simulink library "inp"  (R2021b)
settings: Solver=VariableStepAuto  StartTime=0.0  StopTime=10.0  RelTol=1e-3
undefined symbols (not defined in the file): C_TASK_5MS_S, FALSE, KINP_AcoreReadyToSlp_flg_ovrdflg, KINP_AcoreReadyToSlp_flg_ovrdval, KINP_AllowMovThd_OTA_enum_ovrdflg, KINP_AllowMovThd_OTA_enum_ovrdval, KINP_APSAngleTarget_Deg_ovrdflg, KINP_APSAngleTarget_Deg_ovrdval, KINP_APSDecReq_mps2_ovrdflg, KINP_APSDecReq_mps2_ovrdval, KINP_APSDecReqA_flg_ovrdflg, KINP_APSDecReqA_flg_ovrdval, KINP_APSDFLL_cm_ovrdflg, KINP_APSDFLL_cm_ovrdval, KINP_APSDFLR_cm_ovrdflg, KINP_APSDFLR_cm_ovrdval, KINP_APSDRLL_cm_ovrdflg, KINP_APSDRLL_cm_ovrdval, KINP_APSDRLR_cm_ovrdflg, KINP_APSDRLR_cm_ovrdval, KINP_APSExitCondition_enum_ovrdflg, KINP_APSExitCondition_enum_ovrdval, KINP_APSHWVer_enum_ovrdflg, KINP_APSHWVer_enum_ovrdval, KINP_APSProgressPCT_pct_ovrdflg, KINP_APSProgressPCT_pct_ovrdval, KINP_APSPwrReq_enum_ovrdflg, KINP_APSPwrReq_enum_ovrdval, KINP_APSReq_enum_ovrdflg, KINP_APSReq_enum_ovrdval, KINP_APSRQDisplay_enum_ovrdflg, KINP_APSRQDisplay_enum_ovrdval, KINP_APSRqEPASCtrl_flg_ovrdflg, KINP_APSRqEPASCtrl_flg_ovrdval, KINP_APSShiftPosnReq_enum_ovrdval, KINP_APSShiftPosnReq_enum_ovrflg, KINP_APSSpeedCMD_kph_ovrdval, KINP_APSSpeedCMD_kph_ovrflg, KINP_APSStaSystem_enum_ovrdflg, KINP_APSStaSystem_enum_ovrdval, KINP_APSSWVer_enum_ovrdflg, KINP_APSSWVer_enum_ovrdval, KINP_APSVMCReqA_flg_ovrdval, KINP_APSVMCReqA_flg_ovrflg, KINP_APSVRqEPASCtrl_flg_ovrdflg, KINP_APSVRqEPASCtrl_flg_ovrdval, KINP_AuxBattVolmV_mV_ovrdflg, KINP_AuxBattVolmV_mV_ovrdval, KINP_CAASSta_enum_ovrdflg, KINP_CAASSta_enum_ovrdval, KINP_CAASVMCReqA_flg_ovrdval, KINP_CAASVMCReqA_flg_ovrflg, KINP_CAN1BusOff_flg_ovrdflg, KINP_CAN1BusOff_flg_ovrdval, KINP_CAN2BusOff_flg_ovrdflg, KINP_CAN2BusOff_flg_ovrdval, KINP_CAN3BusOff_flg_ovrdflg, KINP_CAN3BusOff_flg_ovrdval, KINP_CAN4BusOff_flg_ovrdflg, KINP_CAN4BusOff_flg_ovrdval ... (+152)
libraries: FVT_lib x1035, hcu_lib x1
(part 11 of 33)

== system inp/INP/CAN6/CreateBus ==
  inp_CanValid_bus : Inport
  inp_Hal_bus : Inport  Port=2
  UnitConverter_{1..5,14..15,21,23..25,27,42,45..46,52,54,56..60,62..64,67..68,86..87,90,93,96..97} (33 alike) : DataTypeConversion  OutDataTypeStr=boolean
  UnitConverter_{6..10,12..13,35..36,50,70..85,88..89,91..92} (30 alike) : DataTypeConversion  OutDataTypeStr=single
  UnitConverter_{11,16..20,22,26,28..34,37..41,43..44,47..49,51,53,55,61,65..66,69,94..95,98..99} (36 alike) : DataTypeConversion  OutDataTypeStr=uint8
  bus_creator : BusCreator  Inputs=99
  bus_selector : BusSelector  OutputSignals=VINP_CANMsgValidFCM1_flg,VINP_CANMsgValidFCM2_flg,VINP_CANMsgValidFCM3_flg,VINP_CANMsgValidFCM4_flg,VINP_CANMsgValidSRR1_flg
  bus_selector_1 : BusSelector  OutputSignals=VINP_ACCComfortBandLower_mps2,VINP_ACCComfortBandUpper_mps2,VINP_ACCJerkLowerLimit_mps3,VINP_ACCJerkUpperLimit_mps3,VINP_ACCObjDist_m,VINP_ACCObjDstLvl_enum,VINP_ACCObjRelSpd_mps,VINP_ACCRequiredAccel_mps2,VINP_ACCTakeoverReq_flg,VINP_ACCVehHoldReq_flg,VINP_ADASACCSta_enum,VINP_ADASAEBReq_enum,VINP_ADASAEBSta_enum,VINP_ADASCAMSpdLim_enum,VINP_ADASDBSReq_enum,VINP_ADASFCWMute_flg,VINP_ADASFCWSta_enum,VINP_ADASFaultSta_flg,VINP_ADASFltWrnReq_flg,VINP_ADASForceIdle_flg,VINP_ADASISASta_enum,VINP_ADASLDWMute_flg,VINP_ADASLDWSta_enum,VINP_ADASLFCHandsOffWarning_enum,VINP_ADASLFCSta_enum,VINP_ADASLFCWarnSound_enum,VINP_ADASLKASta_enum,VINP_ADASLaneModeL_enum,VINP_ADASLaneModeR_enum,VINP_ADASLanecurveL_raw32,VINP_ADASLanecurveR_raw32,VINP_ADASLanetypeL_enum,VINP_ADASLanetypeR_enum,VINP_ADASSLIFSpdLim_enum,VINP_ADASSLIFSta_enum,VINP_ADASShftPosnReq_enum,VINP_ADASShftPosnReqA_flg,VINP_ADASVehSpdLim_enum,VINP_ADASWarningMsg_enum,VINP_AEBVehHoldReq_flg,VINP_CameraBlockage_flg,VINP_FCM1Checksum_enum,VINP_FCM1LifeCount_enum,VINP_FCMACCmode_enum,VINP_FCMLKAStrToqReq_Nm,VINP_FCMLKATOIAct_enum,VINP_FCMLKATOIFault_flg,VINP_ForceLowBeam_enum,VINP_HazardWarningReq_flg,VINP_ISAWarningMsg_enum,VINP_LKAHODDisplayWarning_flg,VINP_LKAHODSoundWarning_flg,VINP_LVDAACCStatusInformation_flg,VINP_LVDADisabled_flg,VINP_LVDAFailinfo_flg,VINP_LVDAMuteSta_enum,VINP_LVDAWarning_flg,VINP_LeftTurnLightReq_flg,VINP_RightTurnLightReq_flg,VINP_TargetType_enum,VINP_TimeGapLevel_enum,VINP_FCM2CSErr_flg,VINP_FCM2RCErr_flg,VINP_ADBVehDst1Val_enum,VINP_MELaneCurvDervLt_raw32,VINP_MELaneCurvDervLt2_raw32,VINP_MELaneCurvDervRt_raw32,VINP_MELaneCurvDervRt2_raw32,VINP_MELaneCurvLt_raw32,VINP_MELaneCurvLt2_raw32,VINP_MELaneCurvRt_raw32,VINP_MELaneCurvRt2_raw32,VINP_MELaneHeadAngLt_radians,VINP_MELaneHeadAngLt2_radians,VINP_MELaneHeadAngRt_radians,VINP_MELaneHeadAngRt2_radians,VINP_MELanePosLt_m,VINP_MELanePosLt2_m,VINP_MELanePosRt_m,VINP_MELanePosRt2_m,VINP_FCM4CSErr_flg,VINP_FCM4RCErr_flg,VINP_ADASAngCtrlTqWeightGain_pct,VINP_ADASDesStrWhlAngCtrlCmd_Deg,VINP_ADASDrvInputTqBoostAct_flg,VINP_ADASDrvInputTqBoostGain_pct,VINP_ADASMaxAngCtrlOutTqLimit_Nm,VINP_ADASStrWhlAngCtrlStatus_flg,VINP_SRRBSDWarnL_enum,VINP_SRRBSDWarnR_enum,VINP_SRRODASoundL_flg,VINP_SRRODASoundR_flg,VINP_SRRODAWarnL_enum,VINP_SRRODAWarnR_enum
  BINP_outputs : Outport
  wires:
  inp_CanValid_bus/1 -> [inp_CanValid_bus]
  inp_Hal_bus/1 -> [inp_Hal_bus]
  bus_selector/1 -> UnitConverter_1/1  "<VINP_CANMsgValidFCM1_flg>"
  UnitConverter_1/1 -> bus_creator/1  "VINP_CANMsgValidFCM1_flg"
  bus_selector/2 -> UnitConverter_2/1  "<VINP_CANMsgValidFCM2_flg>"
  UnitConverter_2/1 -> bus_creator/2  "VINP_CANMsgValidFCM2_flg"
  bus_selector/3 -> UnitConverter_3/1  "<VINP_CANMsgValidFCM3_flg>"
  UnitConverter_3/1 -> bus_creator/3  "VINP_CANMsgValidFCM3_flg"
  bus_selector/4 -> UnitConverter_4/1  "<VINP_CANMsgValidFCM4_flg>"
  UnitConverter_4/1 -> bus_creator/4  "VINP_CANMsgValidFCM4_flg"
  bus_selector/5 -> UnitConverter_5/1  "<VINP_CANMsgValidSRR1_flg>"
  UnitConverter_5/1 -> bus_creator/5  "VINP_CANMsgValidSRR1_flg"
  bus_selector_1/1 -> UnitConverter_6/1  "<VINP_ACCComfortBandLower_mps2>"
  UnitConverter_6/1 -> bus_creator/6  "VINP_ACCComfortBandLower_mps2"
  bus_selector_1/2 -> UnitConverter_7/1  "<VINP_ACCComfortBandUpper_mps2>"
  UnitConverter_7/1 -> bus_creator/7  "VINP_ACCComfortBandUpper_mps2"
  bus_selector_1/3 -> UnitConverter_8/1  "<VINP_ACCJerkLowerLimit_mps3>"
  UnitConverter_8/1 -> bus_creator/8  "VINP_ACCJerkLowerLimit_mps3"
  bus_selector_1/4 -> UnitConverter_9/1  "<VINP_ACCJerkUpperLimit_mps3>"
  UnitConverter_9/1 -> bus_creator/9  "VINP_ACCJerkUpperLimit_mps3"
  bus_selector_1/5 -> UnitConverter_10/1  "<VINP_ACCObjDist_m>"
  UnitConverter_10/1 -> bus_creator/10  "VINP_ACCObjDist_m"
  bus_selector_1/6 -> UnitConverter_11/1  "<VINP_ACCObjDstLvl_enum>"
  UnitConverter_11/1 -> bus_creator/11  "VINP_ACCObjDstLvl_enum"
  bus_selector_1/7 -> UnitConverter_12/1  "<VINP_ACCObjRelSpd_mps>"
  UnitConverter_12/1 -> bus_creator/12  "VINP_ACCObjRelSpd_mps"
  bus_selector_1/8 -> UnitConverter_13/1  "<VINP_ACCRequiredAccel_mps2>"
  UnitConverter_13/1 -> bus_creator/13  "VINP_ACCRequiredAccel_mps2"
  bus_selector_1/9 -> UnitConverter_14/1  "<VINP_ACCTakeoverReq_flg>"
  UnitConverter_14/1 -> bus_creator/14  "VINP_ACCTakeoverReq_flg"
  bus_selector_1/10 -> UnitConverter_15/1  "<VINP_ACCVehHoldReq_flg>"
  UnitConverter_15/1 -> bus_creator/15  "VINP_ACCVehHoldReq_flg"
  bus_selector_1/11 -> UnitConverter_16/1  "<VINP_ADASACCSta_enum>"
  UnitConverter_16/1 -> bus_creator/16  "VINP_ADASACCSta_enum"
  bus_selector_1/12 -> UnitConverter_17/1  "<VINP_ADASAEBReq_enum>"
  UnitConverter_17/1 -> bus_creator/17  "VINP_ADASAEBReq_enum"
  bus_selector_1/13 -> UnitConverter_18/1  "<VINP_ADASAEBSta_enum>"
  UnitConverter_18/1 -> bus_creator/18  "VINP_ADASAEBSta_enum"
  bus_selector_1/14 -> UnitConverter_19/1  "<VINP_ADASCAMSpdLim_enum>"
  UnitConverter_19/1 -> bus_creator/19  "VINP_ADASCAMSpdLim_enum"
  bus_selector_1/15 -> UnitConverter_20/1  "<VINP_ADASDBSReq_enum>"
  UnitConverter_20/1 -> bus_creator/20  "VINP_ADASDBSReq_enum"
  bus_selector_1/16 -> UnitConverter_21/1  "<VINP_ADASFCWMute_flg>"
  UnitConverter_21/1 -> bus_creator/21  "VINP_ADASFCWMute_flg"
  bus_selector_1/17 -> UnitConverter_22/1  "<VINP_ADASFCWSta_enum>"
  UnitConverter_22/1 -> bus_creator/22  "VINP_ADASFCWSta_enum"
  bus_selector_1/18 -> UnitConverter_23/1  "<VINP_ADASFaultSta_flg>"
  UnitConverter_23/1 -> bus_creator/23  "VINP_ADASFaultSta_flg"
  bus_selector_1/19 -> UnitConverter_24/1  "<VINP_ADASFltWrnReq_flg>"
  UnitConverter_24/1 -> bus_creator/24  "VINP_ADASFltWrnReq_flg"
  bus_selector_1/20 -> UnitConverter_25/1  "<VINP_ADASForceIdle_flg>"
  UnitConverter_25/1 -> bus_creator/25  "VINP_ADASForceIdle_flg"
  bus_selector_1/21 -> UnitConverter_26/1  "<VINP_ADASISASta_enum>"
  UnitConverter_26/1 -> bus_creator/26  "VINP_ADASISASta_enum"
  bus_selector_1/22 -> UnitConverter_27/1  "<VINP_ADASLDWMute_flg>"
  UnitConverter_27/1 -> bus_creator/27  "VINP_ADASLDWMute_flg"
  bus_selector_1/23 -> UnitConverter_28/1  "<VINP_ADASLDWSta_enum>"
  UnitConverter_28/1 -> bus_creator/28  "VINP_ADASLDWSta_enum"
  bus_selector_1/24 -> UnitConverter_29/1  "<VINP_ADASLFCHandsOffWarning_enum>"
  UnitConverter_29/1 -> bus_creator/29  "VINP_ADASLFCHandsOffWarning_enum"
  bus_selector_1/25 -> UnitConverter_30/1  "<VINP_ADASLFCSta_enum>"
  UnitConverter_30/1 -> bus_creator/30  "VINP_ADASLFCSta_enum"
  bus_selector_1/26 -> UnitConverter_31/1  "<VINP_ADASLFCWarnSound_enum>"
  UnitConverter_31/1 -> bus_creator/31  "VINP_ADASLFCWarnSound_enum"
  bus_selector_1/27 -> UnitConverter_32/1  "<VINP_ADASLKASta_enum>"
  UnitConverter_32/1 -> bus_creator/32  "VINP_ADASLKASta_enum"
  bus_selector_1/28 -> UnitConverter_33/1  "<VINP_ADASLaneModeL_enum>"
  UnitConverter_33/1 -> bus_creator/33  "VINP_ADASLaneModeL_enum"
  bus_selector_1/29 -> UnitConverter_34/1  "<VINP_ADASLaneModeR_enum>"
  UnitConverter_34/1 -> bus_creator/34  "VINP_ADASLaneModeR_enum"
  bus_selector_1/30 -> UnitConverter_35/1  "<VINP_ADASLanecurveL_raw32>"
  UnitConverter_35/1 -> bus_creator/35  "VINP_ADASLanecurveL_raw32"
  bus_selector_1/31 -> UnitConverter_36/1  "<VINP_ADASLanecurveR_raw32>"
  UnitConverter_36/1 -> bus_creator/36  "VINP_ADASLanecurveR_raw32"
  bus_selector_1/32 -> UnitConverter_37/1  "<VINP_ADASLanetypeL_enum>"
  UnitConverter_37/1 -> bus_creator/37  "VINP_ADASLanetypeL_enum"
  bus_selector_1/33 -> UnitConverter_38/1  "<VINP_ADASLanetypeR_enum>"
  UnitConverter_38/1 -> bus_creator/38  "VINP_ADASLanetypeR_enum"
  bus_selector_1/34 -> UnitConverter_39/1  "<VINP_ADASSLIFSpdLim_enum>"
  UnitConverter_39/1 -> bus_creator/39  "VINP_ADASSLIFSpdLim_enum"
  bus_selector_1/35 -> UnitConverter_40/1  "<VINP_ADASSLIFSta_enum>"
  UnitConverter_40/1 -> bus_creator/40  "VINP_ADASSLIFSta_enum"
  bus_selector_1/36 -> UnitConverter_41/1  "<VINP_ADASShftPosnReq_enum>"
  UnitConverter_41/1 -> bus_creator/41  "VINP_ADASShftPosnReq_enum"
  bus_selector_1/37 -> UnitConverter_42/1  "<VINP_ADASShftPosnReqA_flg>"
  UnitConverter_42/1 -> bus_creator/42  "VINP_ADASShftPosnReqA_flg"
  bus_selector_1/38 -> UnitConverter_43/1  "<VINP_ADASVehSpdLim_enum>"
  UnitConverter_43/1 -> bus_creator/43  "VINP_ADASVehSpdLim_enum"
  bus_selector_1/39 -> UnitConverter_44/1  "<VINP_ADASWarningMsg_enum>"
  UnitConverter_44/1 -> bus_creator/44  "VINP_ADASWarningMsg_enum"
  bus_selector_1/40 -> UnitConverter_45/1  "<VINP_AEBVehHoldReq_flg>"
  UnitConverter_45/1 -> bus_creator/45  "VINP_AEBVehHoldReq_flg"
  bus_selector_1/41 -> UnitConverter_46/1  "<VINP_CameraBlockage_flg>"
  UnitConverter_46/1 -> bus_creator/46  "VINP_CameraBlockage_flg"
  bus_selector_1/42 -> UnitConverter_47/1  "<VINP_FCM1Checksum_enum>"
  UnitConverter_47/1 -> bus_creator/47  "VINP_FCM1Checksum_enum"
  bus_selector_1/43 -> UnitConverter_48/1  "<VINP_FCM1LifeCount_enum>"
  UnitConverter_48/1 -> bus_creator/48  "VINP_FCM1LifeCount_enum"
  bus_selector_1/44 -> UnitConverter_49/1  "<VINP_FCMACCmode_enum>"
  UnitConverter_49/1 -> bus_creator/49  "VINP_FCMACCmode_enum"
  bus_selector_1/45 -> UnitConverter_50/1  "<VINP_FCMLKAStrToqReq_Nm>"
  UnitConverter_50/1 -> bus_creator/50  "VINP_FCMLKAStrToqReq_Nm"
  bus_selector_1/46 -> UnitConverter_51/1  "<VINP_FCMLKATOIAct_enum>"
  UnitConverter_51/1 -> bus_creator/51  "VINP_FCMLKATOIAct_enum"
  bus_selector_1/47 -> UnitConverter_52/1  "<VINP_FCMLKATOIFault_flg>"
  UnitConverter_52/1 -> bus_creator/52  "VINP_FCMLKATOIFault_flg"
  bus_selector_1/48 -> UnitConverter_53/1  "<VINP_ForceLowBeam_enum>"
  UnitConverter_53/1 -> bus_creator/53  "VINP_ForceLowBeam_enum"
  bus_selector_1/49 -> UnitConverter_54/1  "<VINP_HazardWarningReq_flg>"
  UnitConverter_54/1 -> bus_creator/54  "VINP_HazardWarningReq_flg"
  bus_selector_1/50 -> UnitConverter_55/1  "<VINP_ISAWarningMsg_enum>"
  UnitConverter_55/1 -> bus_creator/55  "VINP_ISAWarningMsg_enum"
  bus_selector_1/51 -> UnitConverter_56/1  "<VINP_LKAHODDisplayWarning_flg>"
  UnitConverter_56/1 -> bus_creator/56  "VINP_LKAHODDisplayWarning_flg"
  bus_selector_1/52 -> UnitConverter_57/1  "<VINP_LKAHODSoundWarning_flg>"
  UnitConverter_57/1 -> bus_creator/57  "VINP_LKAHODSoundWarning_flg"
  bus_selector_1/53 -> UnitConverter_58/1  "<VINP_LVDAACCStatusInformation_flg>"
  UnitConverter_58/1 -> bus_creator/58  "VINP_LVDAACCStatusInformation_flg"
  bus_selector_1/54 -> UnitConverter_59/1  "<VINP_LVDADisabled_flg>"
  UnitConverter_59/1 -> bus_creator/59  "VINP_LVDADisabled_flg"
  bus_selector_1/55 -> UnitConverter_60/1  "<VINP_LVDAFailinfo_flg>"
  UnitConverter_60/1 -> bus_creator/60  "VINP_LVDAFailinfo_flg"
  bus_selector_1/56 -> UnitConverter_61/1  "<VINP_LVDAMuteSta_enum>"
  UnitConverter_61/1 -> bus_creator/61  "VINP_LVDAMuteSta_enum"
  bus_selector_1/57 -> UnitConverter_62/1  "<VINP_LVDAWarning_flg>"
  UnitConverter_62/1 -> bus_creator/62  "VINP_LVDAWarning_flg"
  bus_selector_1/58 -> UnitConverter_63/1  "<VINP_LeftTurnLightReq_flg>"
  UnitConverter_63/1 -> bus_creator/63  "VINP_LeftTurnLightReq_flg"
  bus_selector_1/59 -> UnitConverter_64/1  "<VINP_RightTurnLightReq_flg>"
  UnitConverter_64/1 -> bus_creator/64  "VINP_RightTurnLightReq_flg"
  bus_selector_1/60 -> UnitConverter_65/1  "<VINP_TargetType_enum>"
  UnitConverter_65/1 -> bus_creator/65  "VINP_TargetType_enum"
  bus_selector_1/61 -> UnitConverter_66/1  "<VINP_TimeGapLevel_enum>"
  UnitConverter_66/1 -> bus_creator/66  "VINP_TimeGapLevel_enum"
  bus_selector_1/62 -> UnitConverter_67/1  "<VINP_FCM2CSErr_flg>"
  UnitConverter_67/1 -> bus_creator/67  "VINP_FCM2CSErr_flg"
  bus_selector_1/63 -> UnitConverter_68/1  "<VINP_FCM2RCErr_flg>"
  UnitConverter_68/1 -> bus_creator/68  "VINP_FCM2RCErr_flg"
  bus_selector_1/64 -> UnitConverter_69/1  "<VINP_ADBVehDst1Val_enum>"
  UnitConverter_69/1 -> bus_creator/69  "VINP_ADBVehDst1Val_enum"
  bus_selector_1/65 -> UnitConverter_70/1  "<VINP_MELaneCurvDervLt_raw32>"
  UnitConverter_70/1 -> bus_creator/70  "VINP_MELaneCurvDervLt_raw32"
  bus_selector_1/66 -> UnitConverter_71/1  "<VINP_MELaneCurvDervLt2_raw32>"
  UnitConverter_71/1 -> bus_creator/71  "VINP_MELaneCurvDervLt2_raw32"
  bus_selector_1/67 -> UnitConverter_72/1  "<VINP_MELaneCurvDervRt_raw32>"
  UnitConverter_72/1 -> bus_creator/72  "VINP_MELaneCurvDervRt_raw32"
  bus_selector_1/68 -> UnitConverter_73/1  "<VINP_MELaneCurvDervRt2_raw32>"
  UnitConverter_73/1 -> bus_creator/73  "VINP_MELaneCurvDervRt2_raw32"
  bus_selector_1/69 -> UnitConverter_74/1  "<VINP_MELaneCurvLt_raw32>"
  UnitConverter_74/1 -> bus_creator/74  "VINP_MELaneCurvLt_raw32"
  bus_selector_1/70 -> UnitConverter_75/1  "<VINP_MELaneCurvLt2_raw32>"
  UnitConverter_75/1 -> bus_creator/75  "VINP_MELaneCurvLt2_raw32"
  bus_selector_1/71 -> UnitConverter_76/1  "<VINP_MELaneCurvRt_raw32>"
  UnitConverter_76/1 -> bus_creator/76  "VINP_MELaneCurvRt_raw32"
  bus_selector_1/72 -> UnitConverter_77/1  "<VINP_MELaneCurvRt2_raw32>"
  UnitConverter_77/1 -> bus_creator/77  "VINP_MELaneCurvRt2_raw32"
  bus_selector_1/73 -> UnitConverter_78/1  "<VINP_MELaneHeadAngLt_radians>"
  UnitConverter_78/1 -> bus_creator/78  "VINP_MELaneHeadAngLt_radians"
  bus_selector_1/74 -> UnitConverter_79/1  "<VINP_MELaneHeadAngLt2_radians>"
  UnitConverter_79/1 -> bus_creator/79  "VINP_MELaneHeadAngLt2_radians"
  bus_selector_1/75 -> UnitConverter_80/1  "<VINP_MELaneHeadAngRt_radians>"
  UnitConverter_80/1 -> bus_creator/80  "VINP_MELaneHeadAngRt_radians"
  bus_selector_1/76 -> UnitConverter_81/1  "<VINP_MELaneHeadAngRt2_radians>"
  UnitConverter_81/1 -> bus_creator/81  "VINP_MELaneHeadAngRt2_radians"
  bus_selector_1/77 -> UnitConverter_82/1  "<VINP_MELanePosLt_m>"
  UnitConverter_82/1 -> bus_creator/82  "VINP_MELanePosLt_m"
  bus_selector_1/78 -> UnitConverter_83/1  "<VINP_MELanePosLt2_m>"
  UnitConverter_83/1 -> bus_creator/83  "VINP_MELanePosLt2_m"
  bus_selector_1/79 -> UnitConverter_84/1  "<VINP_MELanePosRt_m>"
  UnitConverter_84/1 -> bus_creator/84  "VINP_MELanePosRt_m"
  bus_selector_1/80 -> UnitConverter_85/1  "<VINP_MELanePosRt2_m>"
  UnitConverter_85/1 -> bus_creator/85  "VINP_MELanePosRt2_m"
  bus_selector_1/81 -> UnitConverter_86/1  "<VINP_FCM4CSErr_flg>"
  UnitConverter_86/1 -> bus_creator/86  "VINP_FCM4CSErr_flg"
  bus_selector_1/82 -> UnitConverter_87/1  "<VINP_FCM4RCErr_flg>"
  UnitConverter_87/1 -> bus_creator/87  "VINP_FCM4RCErr_flg"
  bus_selector_1/83 -> UnitConverter_88/1  "<VINP_ADASAngCtrlTqWeightGain_pct>"
  UnitConverter_88/1 -> bus_creator/88  "VINP_ADASAngCtrlTqWeightGain_pct"
  bus_selector_1/84 -> UnitConverter_89/1  "<VINP_ADASDesStrWhlAngCtrlCmd_Deg>"
  UnitConverter_89/1 -> bus_creator/89  "VINP_ADASDesStrWhlAngCtrlCmd_Deg"
  bus_selector_1/85 -> UnitConverter_90/1  "<VINP_ADASDrvInputTqBoostAct_flg>"
  UnitConverter_90/1 -> bus_creator/90  "VINP_ADASDrvInputTqBoostAct_flg"
  bus_selector_1/86 -> UnitConverter_91/1  "<VINP_ADASDrvInputTqBoostGain_pct>"
  UnitConverter_91/1 -> bus_creator/91  "VINP_ADASDrvInputTqBoostGain_pct"
  bus_selector_1/87 -> UnitConverter_92/1  "<VINP_ADASMaxAngCtrlOutTqLimit_Nm>"
  UnitConverter_92/1 -> bus_creator/92  "VINP_ADASMaxAngCtrlOutTqLimit_Nm"
  bus_selector_1/88 -> UnitConverter_93/1  "<VINP_ADASStrWhlAngCtrlStatus_flg>"
  UnitConverter_93/1 -> bus_creator/93  "VINP_ADASStrWhlAngCtrlStatus_flg"
  bus_selector_1/89 -> UnitConverter_94/1  "<VINP_SRRBSDWarnL_enum>"
  UnitConverter_94/1 -> bus_creator/94  "VINP_SRRBSDWarnL_enum"
  bus_selector_1/90 -> UnitConverter_95/1  "<VINP_SRRBSDWarnR_enum>"
  UnitConverter_95/1 -> bus_creator/95  "VINP_SRRBSDWarnR_enum"
  bus_selector_1/91 -> UnitConverter_96/1  "<VINP_SRRODASoundL_flg>"
  UnitConverter_96/1 -> bus_creator/96  "VINP_SRRODASoundL_flg"
  bus_selector_1/92 -> UnitConverter_97/1  "<VINP_SRRODASoundR_flg>"
  UnitConverter_97/1 -> bus_creator/97  "VINP_SRRODASoundR_flg"
  bus_selector_1/93 -> UnitConverter_98/1  "<VINP_SRRODAWarnL_enum>"
  UnitConverter_98/1 -> bus_creator/98  "VINP_SRRODAWarnL_enum"
  bus_selector_1/94 -> UnitConverter_99/1  "<VINP_SRRODAWarnR_enum>"
  UnitConverter_99/1 -> bus_creator/99  "VINP_SRRODAWarnR_enum"
  [inp_CanValid_bus] -> bus_selector/1
  [inp_Hal_bus] -> bus_selector_1/1
  bus_creator/1 -> BINP_outputs/1

== system inp/INP/CAN6/SignalCheck ==
  inp_CanValid_bus : Inport
  TASK_TIME_S : Inport  Port=2
  BHAL_outputs : Inport  Port=3
  FCM1 : Subsystem
  FCM2 : Subsystem
  FCM3 : Subsystem
  FCM4 : Subsystem
  SRR1 : Subsystem
  bus_creator : BusCreator  Inputs=94
  inp_Hal_bus : Outport
  wires:
  inp_CanValid_bus/1 -> [inp_CanValid_bus]
  TASK_TIME_S/1 -> [TASK_TIME_S]
  BHAL_outputs/1 -> [BHAL_outputs]
  [BHAL_outputs] -> FCM1/1(BHAL_outputs)
  [inp_CanValid_bus] -> FCM1/2(inp_CanValid_bus)
  FCM1/1(VINP_ACCComfortBandLower_mps2) -> [VINP_ACCComfortBandLower_mps2]
  FCM1/2(VINP_ACCComfortBandUpper_mps2) -> [VINP_ACCComfortBandUpper_mps2]
  FCM1/3(VINP_ACCJerkLowerLimit_mps3) -> [VINP_ACCJerkLowerLimit_mps3]
  FCM1/4(VINP_ACCJerkUpperLimit_mps3) -> [VINP_ACCJerkUpperLimit_mps3]
  FCM1/5(VINP_ACCObjDist_m) -> [VINP_ACCObjDist_m]
  FCM1/6(VINP_ACCObjDstLvl_enum) -> [VINP_ACCObjDstLvl_enum]
  FCM1/7(VINP_ACCObjRelSpd_mps) -> [VINP_ACCObjRelSpd_mps]
  FCM1/8(VINP_ACCRequiredAccel_mps2) -> [VINP_ACCRequiredAccel_mps2]
  FCM1/9(VINP_ACCTakeoverReq_flg) -> [VINP_ACCTakeoverReq_flg]
  FCM1/10(VINP_ACCVehHoldReq_flg) -> [VINP_ACCVehHoldReq_flg]
  FCM1/11(VINP_ADASACCSta_enum) -> [VINP_ADASACCSta_enum]
  FCM1/12(VINP_ADASAEBReq_enum) -> [VINP_ADASAEBReq_enum]
  FCM1/13(VINP_ADASAEBSta_enum) -> [VINP_ADASAEBSta_enum]
  FCM1/14(VINP_ADASCAMSpdLim_enum) -> [VINP_ADASCAMSpdLim_enum]
  FCM1/15(VINP_ADASDBSReq_enum) -> [VINP_ADASDBSReq_enum]
  FCM1/16(VINP_ADASFCWMute_flg) -> [VINP_ADASFCWMute_flg]
  FCM1/17(VINP_ADASFCWSta_enum) -> [VINP_ADASFCWSta_enum]
  FCM1/18(VINP_ADASFaultSta_flg) -> [VINP_ADASFaultSta_flg]
  FCM1/19(VINP_ADASFltWrnReq_flg) -> [VINP_ADASFltWrnReq_flg]
  FCM1/20(VINP_ADASForceIdle_flg) -> [VINP_ADASForceIdle_flg]
  FCM1/21(VINP_ADASISASta_enum) -> [VINP_ADASISASta_enum]
  FCM1/22(VINP_ADASLDWMute_flg) -> [VINP_ADASLDWMute_flg]
  FCM1/23(VINP_ADASLDWSta_enum) -> [VINP_ADASLDWSta_enum]
  FCM1/24(VINP_ADASLFCHandsOffWarning_enum) -> [VINP_ADASLFCHandsOffWarning_enum]
  FCM1/25(VINP_ADASLFCSta_enum) -> [VINP_ADASLFCSta_enum]
  FCM1/26(VINP_ADASLFCWarnSound_enum) -> [VINP_ADASLFCWarnSound_enum]
  FCM1/27(VINP_ADASLKASta_enum) -> [VINP_ADASLKASta_enum]
  FCM1/28(VINP_ADASLaneModeL_enum) -> [VINP_ADASLaneModeL_enum]
  FCM1/29(VINP_ADASLaneModeR_enum) -> [VINP_ADASLaneModeR_enum]
  FCM1/30(VINP_ADASLanecurveL_raw32) -> [VINP_ADASLanecurveL_raw32]
  FCM1/31(VINP_ADASLanecurveR_raw32) -> [VINP_ADASLanecurveR_raw32]
  FCM1/32(VINP_ADASLanetypeL_enum) -> [VINP_ADASLanetypeL_enum]
  FCM1/33(VINP_ADASLanetypeR_enum) -> [VINP_ADASLanetypeR_enum]
  FCM1/34(VINP_ADASSLIFSpdLim_enum) -> [VINP_ADASSLIFSpdLim_enum]
  FCM1/35(VINP_ADASSLIFSta_enum) -> [VINP_ADASSLIFSta_enum]
  FCM1/36(VINP_ADASShftPosnReq_enum) -> [VINP_ADASShftPosnReq_enum]
  FCM1/37(VINP_ADASShftPosnReqA_flg) -> [VINP_ADASShftPosnReqA_flg]
  FCM1/38(VINP_ADASVehSpdLim_enum) -> [VINP_ADASVehSpdLim_enum]
  FCM1/39(VINP_ADASWarningMsg_enum) -> [VINP_ADASWarningMsg_enum]
  FCM1/40(VINP_AEBVehHoldReq_flg) -> [VINP_AEBVehHoldReq_flg]
  FCM1/41(VINP_CameraBlockage_flg) -> [VINP_CameraBlockage_flg]
  FCM1/42(VINP_FCM1Checksum_enum) -> [VINP_FCM1Checksum_enum]
  FCM1/43(VINP_FCM1LifeCount_enum) -> [VINP_FCM1LifeCount_enum]
  FCM1/44(VINP_FCMACCmode_enum) -> [VINP_FCMACCmode_enum]
  FCM1/45(VINP_FCMLKAStrToqReq_Nm) -> [VINP_FCMLKAStrToqReq_Nm]
  FCM1/46(VINP_FCMLKATOIAct_enum) -> [VINP_FCMLKATOIAct_enum]
  FCM1/47(VINP_FCMLKATOIFault_flg) -> [VINP_FCMLKATOIFault_flg]
  FCM1/48(VINP_ForceLowBeam_enum) -> [VINP_ForceLowBeam_enum]
  FCM1/49(VINP_HazardWarningReq_flg) -> [VINP_HazardWarningReq_flg]
  FCM1/50(VINP_ISAWarningMsg_enum) -> [VINP_ISAWarningMsg_enum]
  FCM1/51(VINP_LKAHODDisplayWarning_flg) -> [VINP_LKAHODDisplayWarning_flg]
  FCM1/52(VINP_LKAHODSoundWarning_flg) -> [VINP_LKAHODSoundWarning_flg]
  FCM1/53(VINP_LVDAACCStatusInformation_flg) -> [VINP_LVDAACCStatusInformation_flg]
  FCM1/54(VINP_LVDADisabled_flg) -> [VINP_LVDADisabled_flg]
  FCM1/55(VINP_LVDAFailinfo_flg) -> [VINP_LVDAFailinfo_flg]
  FCM1/56(VINP_LVDAMuteSta_enum) -> [VINP_LVDAMuteSta_enum]
  FCM1/57(VINP_LVDAWarning_flg) -> [VINP_LVDAWarning_flg]
  FCM1/58(VINP_LeftTurnLightReq_flg) -> [VINP_LeftTurnLightReq_flg]
  FCM1/59(VINP_RightTurnLightReq_flg) -> [VINP_RightTurnLightReq_flg]
  FCM1/60(VINP_TargetType_enum) -> [VINP_TargetType_enum]
  FCM1/61(VINP_TimeGapLevel_enum) -> [VINP_TimeGapLevel_enum]
  [BHAL_outputs] -> FCM2/1(BHAL_outputs)
  [inp_CanValid_bus] -> FCM2/2(inp_CanValid_bus)
  FCM2/1(VINP_FCM2CSErr_flg) -> [VINP_FCM2CSErr_flg]
  FCM2/2(VINP_FCM2RCErr_flg) -> [VINP_FCM2RCErr_flg]
  FCM2/3(VINP_ADBVehDst1Val_enum) -> [VINP_ADBVehDst1Val_enum]
  [BHAL_outputs] -> FCM3/1(BHAL_outputs)
  [inp_CanValid_bus] -> FCM3/2(inp_CanValid_bus)
  FCM3/1(VINP_MELaneCurvDervLt_raw32) -> [VINP_MELaneCurvDervLt_raw32]
  FCM3/2(VINP_MELaneCurvDervLt2_raw32) -> [VINP_MELaneCurvDervLt2_raw32]
  FCM3/3(VINP_MELaneCurvDervRt_raw32) -> [VINP_MELaneCurvDervRt_raw32]
  FCM3/4(VINP_MELaneCurvDervRt2_raw32) -> [VINP_MELaneCurvDervRt2_raw32]
  FCM3/5(VINP_MELaneCurvLt_raw32) -> [VINP_MELaneCurvLt_raw32]
  FCM3/6(VINP_MELaneCurvLt2_raw32) -> [VINP_MELaneCurvLt2_raw32]
  FCM3/7(VINP_MELaneCurvRt_raw32) -> [VINP_MELaneCurvRt_raw32]
  FCM3/8(VINP_MELaneCurvRt2_raw32) -> [VINP_MELaneCurvRt2_raw32]
  FCM3/9(VINP_MELaneHeadAngLt_radians) -> [VINP_MELaneHeadAngLt_radians]
  FCM3/10(VINP_MELaneHeadAngLt2_radians) -> [VINP_MELaneHeadAngLt2_radians]
  FCM3/11(VINP_MELaneHeadAngRt_radians) -> [VINP_MELaneHeadAngRt_radians]
  FCM3/12(VINP_MELaneHeadAngRt2_radians) -> [VINP_MELaneHeadAngRt2_radians]
  FCM3/13(VINP_MELanePosLt_m) -> [VINP_MELanePosLt_m]
  FCM3/14(VINP_MELanePosLt2_m) -> [VINP_MELanePosLt2_m]
  FCM3/15(VINP_MELanePosRt_m) -> [VINP_MELanePosRt_m]
  FCM3/16(VINP_MELanePosRt2_m) -> [VINP_MELanePosRt2_m]
  [BHAL_outputs] -> FCM4/1(BHAL_outputs)
  [inp_CanValid_bus] -> FCM4/2(inp_CanValid_bus)
  FCM4/1(VINP_FCM4CSErr_flg) -> [VINP_FCM4CSErr_flg]
  FCM4/2(VINP_FCM4RCErr_flg) -> [VINP_FCM4RCErr_flg]
  FCM4/3(VINP_ADASAngCtrlTqWeightGain_pct) -> [VINP_ADASAngCtrlTqWeightGain_pct]
  FCM4/4(VINP_ADASDesStrWhlAngCtrlCmd_Deg) -> [VINP_ADASDesStrWhlAngCtrlCmd_Deg]
  FCM4/5(VINP_ADASDrvInputTqBoostAct_flg) -> [VINP_ADASDrvInputTqBoostAct_flg]
  FCM4/6(VINP_ADASDrvInputTqBoostGain_pct) -> [VINP_ADASDrvInputTqBoostGain_pct]
  FCM4/7(VINP_ADASMaxAngCtrlOutTqLimit_Nm) -> [VINP_ADASMaxAngCtrlOutTqLimit_Nm]
  FCM4/8(VINP_ADASStrWhlAngCtrlStatus_flg) -> [VINP_ADASStrWhlAngCtrlStatus_flg]
  [BHAL_outputs] -> SRR1/1(BHAL_outputs)
  [inp_CanValid_bus] -> SRR1/2(inp_CanValid_bus)
  SRR1/1(VINP_SRRBSDWarnL_enum) -> [VINP_SRRBSDWarnL_enum]
  SRR1/2(VINP_SRRBSDWarnR_enum) -> [VINP_SRRBSDWarnR_enum]
  SRR1/3(VINP_SRRODASoundL_flg) -> [VINP_SRRODASoundL_flg]
  SRR1/4(VINP_SRRODASoundR_flg) -> [VINP_SRRODASoundR_flg]
  SRR1/5(VINP_SRRODAWarnL_enum) -> [VINP_SRRODAWarnL_enum]
  SRR1/6(VINP_SRRODAWarnR_enum) -> [VINP_SRRODAWarnR_enum]
  bus_creator/1 -> inp_Hal_bus/1
  [VINP_ACCComfortBandLower_mps2] -> bus_creator/1
  [VINP_ACCComfortBandUpper_mps2] -> bus_creator/2
  [VINP_ACCJerkLowerLimit_mps3] -> bus_creator/3
  [VINP_ACCJerkUpperLimit_mps3] -> bus_creator/4
  [VINP_ACCObjDist_m] -> bus_creator/5
  [VINP_ACCObjDstLvl_enum] -> bus_creator/6
  [VINP_ACCObjRelSpd_mps] -> bus_creator/7
  [VINP_ACCRequiredAccel_mps2] -> bus_creator/8
  [VINP_ACCTakeoverReq_flg] -> bus_creator/9
  [VINP_ACCVehHoldReq_flg] -> bus_creator/10
  [VINP_ADASACCSta_enum] -> bus_creator/11
  [VINP_ADASAEBReq_enum] -> bus_creator/12
  [VINP_ADASAEBSta_enum] -> bus_creator/13
  [VINP_ADASCAMSpdLim_enum] -> bus_creator/14
  [VINP_ADASDBSReq_enum] -> bus_creator/15
  [VINP_ADASFCWMute_flg] -> bus_creator/16
  [VINP_ADASFCWSta_enum] -> bus_creator/17
  [VINP_ADASFaultSta_flg] -> bus_creator/18
  [VINP_ADASFltWrnReq_flg] -> bus_creator/19
  [VINP_ADASForceIdle_flg] -> bus_creator/20
  [VINP_ADASISASta_enum] -> bus_creator/21
  [VINP_ADASLDWMute_flg] -> bus_creator/22
  [VINP_ADASLDWSta_enum] -> bus_creator/23
  [VINP_ADASLFCHandsOffWarning_enum] -> bus_creator/24
  [VINP_ADASLFCSta_enum] -> bus_creator/25
  [VINP_ADASLFCWarnSound_enum] -> bus_creator/26
  [VINP_ADASLKASta_enum] -> bus_creator/27
  [VINP_ADASLaneModeL_enum] -> bus_creator/28
  [VINP_ADASLaneModeR_enum] -> bus_creator/29
  [VINP_ADASLanecurveL_raw32] -> bus_creator/30
  [VINP_ADASLanecurveR_raw32] -> bus_creator/31
  [VINP_ADASLanetypeL_enum] -> bus_creator/32
  [VINP_ADASLanetypeR_enum] -> bus_creator/33
  [VINP_ADASSLIFSpdLim_enum] -> bus_creator/34
  [VINP_ADASSLIFSta_enum] -> bus_creator/35
  [VINP_ADASShftPosnReq_enum] -> bus_creator/36
  [VINP_ADASShftPosnReqA_flg] -> bus_creator/37
  [VINP_ADASVehSpdLim_enum] -> bus_creator/38
  [VINP_ADASWarningMsg_enum] -> bus_creator/39
  [VINP_AEBVehHoldReq_flg] -> bus_creator/40
  [VINP_CameraBlockage_flg] -> bus_creator/41
  [VINP_FCM1Checksum_enum] -> bus_creator/42
  [VINP_FCM1LifeCount_enum] -> bus_creator/43
  [VINP_FCMACCmode_enum] -> bus_creator/44
  [VINP_FCMLKAStrToqReq_Nm] -> bus_creator/45
  [VINP_FCMLKATOIAct_enum] -> bus_creator/46
  [VINP_FCMLKATOIFault_flg] -> bus_creator/47
  [VINP_ForceLowBeam_enum] -> bus_creator/48
  [VINP_HazardWarningReq_flg] -> bus_creator/49
  [VINP_ISAWarningMsg_enum] -> bus_creator/50
  [VINP_LKAHODDisplayWarning_flg] -> bus_creator/51
  [VINP_LKAHODSoundWarning_flg] -> bus_creator/52
  [VINP_LVDAACCStatusInformation_flg] -> bus_creator/53
  [VINP_LVDADisabled_flg] -> bus_creator/54
  [VINP_LVDAFailinfo_flg] -> bus_creator/55
  [VINP_LVDAMuteSta_enum] -> bus_creator/56
  [VINP_LVDAWarning_flg] -> bus_creator/57
  [VINP_LeftTurnLightReq_flg] -> bus_creator/58
  [VINP_RightTurnLightReq_flg] -> bus_creator/59
  [VINP_TargetType_enum] -> bus_creator/60
  [VINP_TimeGapLevel_enum] -> bus_creator/61
  [VINP_FCM2CSErr_flg] -> bus_creator/62
  [VINP_FCM2RCErr_flg] -> bus_creator/63
  [VINP_ADBVehDst1Val_enum] -> bus_creator/64
  [VINP_MELaneCurvDervLt_raw32] -> bus_creator/65
  [VINP_MELaneCurvDervLt2_raw32] -> bus_creator/66
  [VINP_MELaneCurvDervRt_raw32] -> bus_creator/67
  [VINP_MELaneCurvDervRt2_raw32] -> bus_creator/68
  [VINP_MELaneCurvLt_raw32] -> bus_creator/69
  [VINP_MELaneCurvLt2_raw32] -> bus_creator/70
  [VINP_MELaneCurvRt_raw32] -> bus_creator/71
  [VINP_MELaneCurvRt2_raw32] -> bus_creator/72
  [VINP_MELaneHeadAngLt_radians] -> bus_creator/73
  [VINP_MELaneHeadAngLt2_radians] -> bus_creator/74
  [VINP_MELaneHeadAngRt_radians] -> bus_creator/75
  [VINP_MELaneHeadAngRt2_radians] -> bus_creator/76
  [VINP_MELanePosLt_m] -> bus_creator/77
  [VINP_MELanePosLt2_m] -> bus_creator/78
  [VINP_MELanePosRt_m] -> bus_creator/79
  [VINP_MELanePosRt2_m] -> bus_creator/80
  [VINP_FCM4CSErr_flg] -> bus_creator/81
  [VINP_FCM4RCErr_flg] -> bus_creator/82
  [VINP_ADASAngCtrlTqWeightGain_pct] -> bus_creator/83
  [VINP_ADASDesStrWhlAngCtrlCmd_Deg] -> bus_creator/84
  [VINP_ADASDrvInputTqBoostAct_flg] -> bus_creator/85
  [VINP_ADASDrvInputTqBoostGain_pct] -> bus_creator/86
  [VINP_ADASMaxAngCtrlOutTqLimit_Nm] -> bus_creator/87
  [VINP_ADASStrWhlAngCtrlStatus_flg] -> bus_creator/88
  [VINP_SRRBSDWarnL_enum] -> bus_creator/89
  [VINP_SRRBSDWarnR_enum] -> bus_creator/90
  [VINP_SRRODASoundL_flg] -> bus_creator/91
  [VINP_SRRODASoundR_flg] -> bus_creator/92
  [VINP_SRRODAWarnL_enum] -> bus_creator/93
  [VINP_SRRODAWarnR_enum] -> bus_creator/94

== system inp/INP/DDM/Subsystem13 ==
  In1 : Inport
  Constant : Constant  Value=KINP_ClearDTCcmd_flg_ovrdval
  Constant1 : Constant  Value=KINP_ClearDTCcmd_flg_ovrdflg
  Switch : Switch  Criteria=u2 ~= 0
  Out1 : Outport
  wires:
  Constant1/1 -> Switch/2
  Constant/1 -> Switch/1
  Switch/1 -> Out1/1
  In1/1 -> Switch/3

== system inp/INP/DKC/Subsystem1 ==
  In1 : Inport
  Constant : Constant  Value=KINP_NFCLidASta_flg_ovrdval
  Constant1 : Constant  Value=KINP_NFCLidASta_flg_ovrdflg
  Switch : Switch  Criteria=u2 ~= 0
  Out1 : Outport
  wires:
  Constant1/1 -> Switch/2
  Constant/1 -> Switch/1
  Switch/1 -> Out1/1
  In1/1 -> Switch/3

== system inp/INP/DKC/Subsystem10 ==
  In1 : Inport
  Constant : Constant  Value=KINP_NFCDoorSta_flg_ovrdval
  Constant1 : Constant  Value=KINP_NFCDoorSta_flg_ovrdflg
  Switch : Switch  Criteria=u2 ~= 0
  Out1 : Outport
  wires:
  Constant1/1 -> Switch/2
  Constant/1 -> Switch/1
  Switch/1 -> Out1/1
  In1/1 -> Switch/3

== system inp/INP/DKC/Subsystem2 ==
  In1 : Inport
  Constant : Constant  Value=KINP_KeyFobAreaU16_enum_ovrdval
  Constant1 : Constant  Value=KINP_KeyFobAreaU16_enum_ovrdflg
  Switch : Switch  Criteria=u2 ~= 0
  Out1 : Outport
  wires:
  Constant1/1 -> Switch/2
  Constant/1 -> Switch/1
  Switch/1 -> Out1/1
  In1/1 -> Switch/3

== system inp/INP/DKC/Subsystem3 ==
  In1 : Inport
  Constant : Constant  Value=KINP_UIDButtonCmd_enum_ovrdval
  Constant1 : Constant  Value=KINP_UIDButtonCmd_enum_ovrdflg
  Switch : Switch  Criteria=u2 ~= 0
  Out1 : Outport
  wires:
  Constant1/1 -> Switch/2
  Constant/1 -> Switch/1
  Switch/1 -> Out1/1
  In1/1 -> Switch/3

== system inp/INP/GPIO/Analog ==
  BHAL_outputs : Inport
  TASK_TIME_S : Inport  Port=2
  AccelPedal1Vol_V : FVT_lib/inp/ad_signal_template  SystemSampleTime=-1  VariantActivationTime=update diagram  Latency=0  AutoFrameSizeCalculation=off
      link override defval: Value=KINP_AccelPedal1Vol_V_defval
      link override fftdec: Value=KINP_AccelPedal1Vol_V_fftdec
      link override fftinc: Value=KINP_AccelPedal1Vol_V_fftinc
      link override fftlim: Value=KINP_AccelPedal1Vol_V_fftlim
      link override limlow: Value=KINP_AccelPedal1Vol_V_limlow
      link override limupr: Value=KINP_AccelPedal1Vol_V_limupr
      link override ovrdflg: Value=KINP_AccelPedal1Vol_V_ovrdflg
      link override ovrdval: Value=KINP_AccelPedal1Vol_V_ovrdval
      link override srvcflg: Value=KINP_AccelPedal1Vol_V_srvcflg
      link override srvcval: Value=KINP_AccelPedal1Vol_V_srvcval
      link override tcfilt: Value=KINP_AccelPedal1Vol_V_tcfilt
  AccelPedal2Vol_V : FVT_lib/inp/ad_signal_template  SystemSampleTime=-1  VariantActivationTime=update diagram  Latency=0  AutoFrameSizeCalculation=off
      link override defval: Value=KINP_AccelPedal2Vol_V_defval
      link override fftdec: Value=KINP_AccelPedal2Vol_V_fftdec
      link override fftinc: Value=KINP_AccelPedal2Vol_V_fftinc
      link override fftlim: Value=KINP_AccelPedal2Vol_V_fftlim
      link override limlow: Value=KINP_AccelPedal2Vol_V_limlow
      link override limupr: Value=KINP_AccelPedal2Vol_V_limupr
      link override ovrdflg: Value=KINP_AccelPedal2Vol_V_ovrdflg
      link override ovrdval: Value=KINP_AccelPedal2Vol_V_ovrdval
      link override srvcflg: Value=KINP_AccelPedal2Vol_V_srvcflg
      link override srvcval: Value=KINP_AccelPedal2Vol_V_srvcval
      link override tcfilt: Value=KINP_AccelPedal2Vol_V_tcfilt
  Bus Selector : BusSelector  OutputSignals=VHAL_AccelPedal1Vol_V
  Bus Selector1 : BusSelector  OutputSignals=VHAL_AccelPedal2Vol_V
  Constant{,1..3} (4 alike) : Constant  Value=FALSE
  VINP_AccelPedal1VolShortHigh_enum : Outport
  VINP_AccelPedal1VolShortLow_enum : Outport  Port=2
  VINP_AccelPedal1Vol_V : Outport  Port=3
  VINP_AccelPedal1VolValid_flg : Outport  Port=4
  VINP_AccelPedal2VolShortHigh_enum : Outport  Port=5
  VINP_AccelPedal2VolShortLow_enum : Outport  Port=6
  VINP_AccelPedal2Vol_V : Outport  Port=7
  VINP_AccelPedal2VolValid_flg : Outport  Port=8
  wires:
  BHAL_outputs/1 -> [BHAL_outputs]
  TASK_TIME_S/1 -> [TASK_TIME_S]
  AccelPedal1Vol_V/1 -> VINP_AccelPedal1VolShortHigh_enum/1  "VINP_AccelPedal1VolShortHigh_enum"
  AccelPedal1Vol_V/2 -> VINP_AccelPedal1VolShortLow_enum/1  "VINP_AccelPedal1VolShortLow_enum"
  AccelPedal1Vol_V/3 -> VINP_AccelPedal1Vol_V/1  "VINP_AccelPedal1Vol_V"
  AccelPedal1Vol_V/4 -> VINP_AccelPedal1VolValid_flg/1  "VINP_AccelPedal1VolValid_flg"
  AccelPedal2Vol_V/1 -> VINP_AccelPedal2VolShortHigh_enum/1  "VINP_AccelPedal2VolShortHigh_enum"
  AccelPedal2Vol_V/2 -> VINP_AccelPedal2VolShortLow_enum/1  "VINP_AccelPedal2VolShortLow_enum"
  AccelPedal2Vol_V/3 -> VINP_AccelPedal2Vol_V/1  "VINP_AccelPedal2Vol_V"
  AccelPedal2Vol_V/4 -> VINP_AccelPedal2VolValid_flg/1  "VINP_AccelPedal2VolValid_flg"
  [TASK_TIME_S] -> AccelPedal1Vol_V/4
  Constant1/1 -> AccelPedal1Vol_V/3
  Constant/1 -> AccelPedal1Vol_V/2
  [BHAL_outputs] -> Bus Selector/1
  Bus Selector/1 -> AccelPedal1Vol_V/1  "<VHAL_AccelPedal1Vol_V>"
  Bus Selector1/1 -> AccelPedal2Vol_V/1  "<VHAL_AccelPedal2Vol_V>"
  [BHAL_outputs] -> Bus Selector1/1
  Constant2/1 -> AccelPedal2Vol_V/2
  Constant3/1 -> AccelPedal2Vol_V/3
  [TASK_TIME_S] -> AccelPedal2Vol_V/4

== system inp/INP/GPIO/Digital ==
  BHAL_outputs : Inport
  BrakeLampSW : FVT_lib/inp/di_signal_template  SystemSampleTime=-1  VariantActivationTime=update diagram  Latency=0  AutoFrameSizeCalculation=off
      link override debdec: Value=KINP_BrakeLampSW_flg_debdec
      link override debinc: Value=KINP_BrakeLampSW_flg_debinc
      link override deblim: Value=KINP_BrakeLampSW_flg_deblim
      link override inverse: Value=KINP_BrakeLampSW_flg_inverse
      link override ovrdflg: Value=KINP_BrakeLampSW_flg_ovrdflg
      link override ovrdval: Value=KINP_BrakeLampSW_flg_ovrdval
      link override srvcflg: Value=KINP_BrakeLampSW_flg_srvcflg
      link override srvcval: Value=KINP_BrakeLampSW_flg_srvcval
  BrakeSWGPIO : FVT_lib/inp/di_signal_template  SystemSampleTime=-1  VariantActivationTime=update diagram  Latency=0  AutoFrameSizeCalculation=off
      link override debdec: Value=KINP_BrakeSWGPIO_flg_debdec
      link override debinc: Value=KINP_BrakeSWGPIO_flg_debinc
      link override deblim: Value=KINP_BrakeSWGPIO_flg_deblim
      link override inverse: Value=KINP_BrakeSWGPIO_flg_inverse
      link override ovrdflg: Value=KINP_BrakeSWGPIO_flg_ovrdflg
      link override ovrdval: Value=KINP_BrakeSWGPIO_flg_ovrdval
      link override srvcflg: Value=KINP_BrakeSWGPIO_flg_srvcflg
      link override srvcval: Value=KINP_BrakeSWGPIO_flg_srvcval
  CentralDoorLockSW : FVT_lib/inp/di_signal_template  SystemSampleTime=-1  VariantActivationTime=update diagram  Latency=0  AutoFrameSizeCalculation=off
      link override debdec: Value=KINP_CentralDoorLockSW_flg_debdec
      link override debinc: Value=KINP_CentralDoorLockSW_flg_debinc
      link override deblim: Value=KINP_CentralDoorLockSW_flg_deblim
      link override inverse: Value=KINP_CentralDoorLockSW_flg_inverse
      link override ovrdflg: Value=KINP_CentralDoorLockSW_flg_ovrdflg
      link override ovrdval: Value=KINP_CentralDoorLockSW_flg_ovrdval
      link override srvcflg: Value=KINP_CentralDoorLockSW_flg_srvcflg
      link override srvcval: Value=KINP_CentralDoorLockSW_flg_srvcval
  CrashSignalGPIO : FVT_lib/inp/di_signal_template  SystemSampleTime=-1  VariantActivationTime=update diagram  Latency=0  AutoFrameSizeCalculation=off
      link override debdec: Value=KINP_CrashSignalGPIO_flg_debdec
      link override debinc: Value=KINP_CrashSignalGPIO_flg_debinc
      link override deblim: Value=KINP_CrashSignalGPIO_flg_deblim
      link override inverse: Value=KINP_CrashSignalGPIO_flg_inverse
      link override ovrdflg: Value=KINP_CrashSignalGPIO_flg_ovrdflg
      link override ovrdval: Value=KINP_CrashSignalGPIO_flg_ovrdval
      link override srvcflg: Value=KINP_CrashSignalGPIO_flg_srvcflg
      link override srvcval: Value=KINP_CrashSignalGPIO_flg_srvcval
  DrDoorSW : FVT_lib/inp/di_signal_template  SystemSampleTime=-1  VariantActivationTime=update diagram  Latency=0  AutoFrameSizeCalculation=off
      link override debdec: Value=KINP_DrDoorSW_flg_debdec
      link override debinc: Value=KINP_DrDoorSW_flg_debinc
      link override deblim: Value=KINP_DrDoorSW_flg_deblim
      link override inverse: Value=KINP_DrDoorSW_flg_inverse
      link override ovrdflg: Value=KINP_DrDoorSW_flg_ovrdflg
      link override ovrdval: Value=KINP_DrDoorSW_flg_ovrdval
      link override srvcflg: Value=KINP_DrDoorSW_flg_srvcflg
      link override srvcval: Value=KINP_DrDoorSW_flg_srvcval
  HazardSW : FVT_lib/inp/di_signal_template  SystemSampleTime=-1  VariantActivationTime=update diagram  Latency=0  AutoFrameSizeCalculation=off
      link override debdec: Value=KINP_HazardSW_flg_debdec
      link override debinc: Value=KINP_HazardSW_flg_debinc
      link override deblim: Value=KINP_HazardSW_flg_deblim
      link override inverse: Value=KINP_HazardSW_flg_inverse
      link override ovrdflg: Value=KINP_HazardSW_flg_ovrdflg
      link override ovrdval: Value=KINP_HazardSW_flg_ovrdval
      link override srvcflg: Value=KINP_HazardSW_flg_srvcflg
      link override srvcval: Value=KINP_HazardSW_flg_srvcval
  HoodSW : FVT_lib/inp/di_signal_template  SystemSampleTime=-1  VariantActivationTime=update diagram  Latency=0  AutoFrameSizeCalculation=off
      link override debdec: Value=KINP_HoodSW_flg_debdec
      link override debinc: Value=KINP_HoodSW_flg_debinc
      link override deblim: Value=KINP_HoodSW_flg_deblim
      link override inverse: Value=KINP_HoodSW_flg_inverse
      link override ovrdflg: Value=KINP_HoodSW_flg_ovrdflg
      link override ovrdval: Value=KINP_HoodSW_flg_ovrdval
      link override srvcflg: Value=KINP_HoodSW_flg_srvcflg
      link override srvcval: Value=KINP_HoodSW_flg_srvcval
  PsDoorSW : FVT_lib/inp/di_signal_template  SystemSampleTime=-1  VariantActivationTime=update diagram  Latency=0  AutoFrameSizeCalculation=off
      link override debdec: Value=KINP_PsDoorSW_flg_debdec
      link override debinc: Value=KINP_PsDoorSW_flg_debinc
      link override deblim: Value=KINP_PsDoorSW_flg_deblim
      link override inverse: Value=KINP_PsDoorSW_flg_inverse
      link override ovrdflg: Value=KINP_PsDoorSW_flg_ovrdflg
      link override ovrdval: Value=KINP_PsDoorSW_flg_ovrdval
      link override srvcflg: Value=KINP_PsDoorSW_flg_srvcflg
      link override srvcval: Value=KINP_PsDoorSW_flg_srvcval
  RLDoorSW : FVT_lib/inp/di_signal_template  SystemSampleTime=-1  VariantActivationTime=update diagram  Latency=0  AutoFrameSizeCalculation=off
      link override debdec: Value=KINP_RLDoorSW_flg_debdec
      link override debinc: Value=KINP_RLDoorSW_flg_debinc
      link override deblim: Value=KINP_RLDoorSW_flg_deblim
      link override inverse: Value=KINP_RLDoorSW_flg_inverse
      link override ovrdflg: Value=KINP_RLDoorSW_flg_ovrdflg
      link override ovrdval: Value=KINP_RLDoorSW_flg_ovrdval
      link override srvcflg: Value=KINP_RLDoorSW_flg_srvcflg
      link override srvcval: Value=KINP_RLDoorSW_flg_srvcval
  RRDoorSW : FVT_lib/inp/di_signal_template  SystemSampleTime=-1  VariantActivationTime=update diagram  Latency=0  AutoFrameSizeCalculation=off
      link override debdec: Value=KINP_RRDoorSW_flg_debdec
      link override debinc: Value=KINP_RRDoorSW_flg_debinc
      link override deblim: Value=KINP_RRDoorSW_flg_deblim
      link override inverse: Value=KINP_RRDoorSW_flg_inverse
      link override ovrdflg: Value=KINP_RRDoorSW_flg_ovrdflg
      link override ovrdval: Value=KINP_RRDoorSW_flg_ovrdval
      link override srvcflg: Value=KINP_RRDoorSW_flg_srvcflg
      link override srvcval: Value=KINP_RRDoorSW_flg_srvcval
  SeatSW : FVT_lib/inp/di_signal_template  SystemSampleTime=-1  VariantActivationTime=update diagram  Latency=0  AutoFrameSizeCalculation=off
      link override debdec: Value=KINP_SeatSW_flg_debdec
      link override debinc: Value=KINP_SeatSW_flg_debinc
      link override deblim: Value=KINP_SeatSW_flg_deblim
      link override inverse: Value=KINP_SeatSW_flg_inverse
      link override ovrdflg: Value=KINP_SeatSW_flg_ovrdflg
      link override ovrdval: Value=KINP_SeatSW_flg_ovrdval
      link override srvcflg: Value=KINP_SeatSW_flg_srvcflg
      link override srvcval: Value=KINP_SeatSW_flg_srvcval
  TailgateSW : FVT_lib/inp/di_signal_template  SystemSampleTime=-1  VariantActivationTime=update diagram  Latency=0  AutoFrameSizeCalculation=off
      link override debdec: Value=KINP_TailgateSW_flg_debdec
      link override debinc: Value=KINP_TailgateSW_flg_debinc
      link override deblim: Value=KINP_TailgateSW_flg_deblim
      link override inverse: Value=KINP_TailgateSW_flg_inverse
      link override ovrdflg: Value=KINP_TailgateSW_flg_ovrdflg
      link override ovrdval: Value=KINP_TailgateSW_flg_ovrdval
      link override srvcflg: Value=KINP_TailgateSW_flg_srvcflg
      link override srvcval: Value=KINP_TailgateSW_flg_srvcval
  TrunkHanSW : FVT_lib/inp/di_signal_template  SystemSampleTime=-1  VariantActivationTime=update diagram  Latency=0  AutoFrameSizeCalculation=off
      link override debdec: Value=KINP_TrunkHanSW_flg_debdec
      link override debinc: Value=KINP_TrunkHanSW_flg_debinc
      link override deblim: Value=KINP_TrunkHanSW_flg_deblim
      link override inverse: Value=KINP_TrunkHanSW_flg_inverse
      link override ovrdflg: Value=KINP_TrunkHanSW_flg_ovrdflg
      link override ovrdval: Value=KINP_TrunkHanSW_flg_ovrdval
      link override srvcflg: Value=KINP_TrunkHanSW_flg_srvcflg
      link override srvcval: Value=KINP_TrunkHanSW_flg_srvcval
  slr_VINP_BrakeLampSW_flg : BusSelector  OutputSignals=VHAL_BrakeLampSW_flg
  slr_VINP_BrakeSWGPIO_flg : BusSelector  OutputSignals=VHAL_BrakeSWGPIO_flg
  slr_VINP_CentralDoorLockSW_flg : BusSelector  OutputSignals=VHAL_CentralDoorLockSW_flg
  slr_VINP_CrashSignalGPIO_flg : BusSelector  OutputSignals=VHAL_CrashSignalGPIO_flg
  slr_VINP_DrDoorSW_flg : BusSelector  OutputSignals=VHAL_DrDoorSW_flg
  slr_VINP_HazardSW_flg : BusSelector  OutputSignals=VHAL_HazardSW_flg
  slr_VINP_HoodSW_flg : BusSelector  OutputSignals=VHAL_HoodSW_flg
  slr_VINP_PsDoorSW_flg : BusSelector  OutputSignals=VHAL_PsDoorSW_flg
  slr_VINP_RLDoorSW_flg : BusSelector  OutputSignals=VHAL_RLDoorSW_flg
  slr_VINP_RRDoorSW_flg : BusSelector  OutputSignals=VHAL_RRDoorSW_flg
  slr_VINP_SeatSW_flg : BusSelector  OutputSignals=VHAL_SeatSW_flg
  slr_VINP_TailgateSW_flg : BusSelector  OutputSignals=VHAL_TailgateSW_flg
  slr_VINP_TrunkHanSW_flg : BusSelector  OutputSignals=VHAL_TrunkHanSW_flg
  VINP_BrakeSWGPIO_flg : Outport
  VINP_HoodSW_flg : Outport  Port=2
  VINP_TailgateSW_flg : Outport  Port=3
  VINP_DrDoorSW_flg : Outport  Port=4
  VINP_PsDoorSW_flg : Outport  Port=5
  VINP_RRDoorSW_flg : Outport  Port=6
  VINP_RLDoorSW_flg : Outport  Port=7
  VINP_CentralDoorLockSW_flg : Outport  Port=8
  VINP_HazardSW_flg : Outport  Port=9
  VINP_BrakeLampSW_flg : Outport  Port=10
  VINP_TrunkHanSW_flg : Outport  Port=11
  VINP_SeatSW_flg : Outport  Port=12
  VINP_CrashSignalGPIO_flg : Outport  Port=13
  wires:
  BHAL_outputs/1 -> [BHAL_outputs]
  BrakeSWGPIO/1 -> VINP_BrakeSWGPIO_flg/1  "VINP_BrakeSWGPIO_flg"
  [BHAL_outputs] -> slr_VINP_BrakeSWGPIO_flg/1
  slr_VINP_BrakeSWGPIO_flg/1 -> BrakeSWGPIO/1  "<VHAL_BrakeSWGPIO_flg>"
  HoodSW/1 -> VINP_HoodSW_flg/1  "VINP_HoodSW_flg"
  [BHAL_outputs] -> slr_VINP_HoodSW_flg/1
  slr_VINP_HoodSW_flg/1 -> HoodSW/1  "<VHAL_HoodSW_flg>"
  TailgateSW/1 -> VINP_TailgateSW_flg/1  "VINP_TailgateSW_flg"
  [BHAL_outputs] -> slr_VINP_TailgateSW_flg/1
  slr_VINP_TailgateSW_flg/1 -> TailgateSW/1  "<VHAL_TailgateSW_flg>"
  DrDoorSW/1 -> VINP_DrDoorSW_flg/1  "VINP_DrDoorSW_flg"
  [BHAL_outputs] -> slr_VINP_DrDoorSW_flg/1
  slr_VINP_DrDoorSW_flg/1 -> DrDoorSW/1  "<VHAL_DrDoorSW_flg>"
  PsDoorSW/1 -> VINP_PsDoorSW_flg/1  "VINP_PsDoorSW_flg"
  [BHAL_outputs] -> slr_VINP_PsDoorSW_flg/1
  slr_VINP_PsDoorSW_flg/1 -> PsDoorSW/1  "<VHAL_PsDoorSW_flg>"
  RRDoorSW/1 -> VINP_RRDoorSW_flg/1  "VINP_RRDoorSW_flg"
  [BHAL_outputs] -> slr_VINP_RRDoorSW_flg/1
  slr_VINP_RRDoorSW_flg/1 -> RRDoorSW/1  "<VHAL_RRDoorSW_flg>"
  RLDoorSW/1 -> VINP_RLDoorSW_flg/1  "VINP_RLDoorSW_flg"
  [BHAL_outputs] -> slr_VINP_RLDoorSW_flg/1
  slr_VINP_RLDoorSW_flg/1 -> RLDoorSW/1  "<VHAL_RLDoorSW_flg>"
  CentralDoorLockSW/1 -> VINP_CentralDoorLockSW_flg/1  "VINP_CentralDoorLockSW_flg"
  [BHAL_outputs] -> slr_VINP_CentralDoorLockSW_flg/1
  slr_VINP_CentralDoorLockSW_flg/1 -> CentralDoorLockSW/1  "<VHAL_CentralDoorLockSW_flg>"
  HazardSW/1 -> VINP_HazardSW_flg/1  "VINP_HazardSW_flg"
  [BHAL_outputs] -> slr_VINP_HazardSW_flg/1
  slr_VINP_HazardSW_flg/1 -> HazardSW/1  "<VHAL_HazardSW_flg>"
  BrakeLampSW/1 -> VINP_BrakeLampSW_flg/1  "VINP_BrakeLampSW_flg"
  [BHAL_outputs] -> slr_VINP_BrakeLampSW_flg/1
  slr_VINP_BrakeLampSW_flg/1 -> BrakeLampSW/1  "<VHAL_BrakeLampSW_flg>"
  TrunkHanSW/1 -> VINP_TrunkHanSW_flg/1  "VINP_TrunkHanSW_flg"
  [BHAL_outputs] -> slr_VINP_TrunkHanSW_flg/1
  slr_VINP_TrunkHanSW_flg/1 -> TrunkHanSW/1  "<VHAL_TrunkHanSW_flg>"
  SeatSW/1 -> VINP_SeatSW_flg/1  "VINP_SeatSW_flg"
  [BHAL_outputs] -> slr_VINP_SeatSW_flg/1
  slr_VINP_SeatSW_flg/1 -> SeatSW/1  "<VHAL_SeatSW_flg>"
  [BHAL_outputs] -> slr_VINP_CrashSignalGPIO_flg/1
  slr_VINP_CrashSignalGPIO_flg/1 -> CrashSignalGPIO/1  "<VHAL_CrashSignalGPIO_flg>"
  CrashSignalGPIO/1 -> VINP_CrashSignalGPIO_flg/1  "VINP_CrashSignalGPIO_flg"

== system inp/INP/IMU/Subsystem1 ==
  In1 : Inport
  Constant : Constant  Value=KINP_MemOffsetGyroY_raw16_ovrdval
  Constant1 : Constant  Value=KINP_MemOffsetGyroY_raw16_ovrdflg
  Switch : Switch  Criteria=u2 ~= 0
  Out1 : Outport
  wires:
  Switch/1 -> Out1/1
  Constant/1 -> Switch/1
  Constant1/1 -> Switch/2
  In1/1 -> Switch/3

== system inp/INP/IMU/Subsystem10 ==
  In1 : Inport
  Constant : Constant  Value=KINP_SensingAccZ_raw16_ovrdval
  Constant1 : Constant  Value=KINP_SensingAccZ_raw16_ovrdflg
  Switch : Switch  Criteria=u2 ~= 0
  Out1 : Outport
  wires:
  Constant1/1 -> Switch/2
  Constant/1 -> Switch/1
  Switch/1 -> Out1/1
  In1/1 -> Switch/3

== system inp/INP/IMU/Subsystem11 ==
  In1 : Inport
  Constant : Constant  Value=KINP_SensingAccY_raw16_ovrdval
  Constant1 : Constant  Value=KINP_SensingAccY_raw16_ovrdflg
  Switch : Switch  Criteria=u2 ~= 0
  Out1 : Outport
  wires:
  Switch/1 -> Out1/1
  Constant/1 -> Switch/1
  Constant1/1 -> Switch/2
  In1/1 -> Switch/3

== system inp/INP/IMU/Subsystem15 ==
  In1 : Inport
  Constant : Constant  Value=KINP_MemOffsetGyroX_raw16_ovrdval
  Constant1 : Constant  Value=KINP_MemOffsetGyroX_raw16_ovrdflg
  Switch : Switch  Criteria=u2 ~= 0
  Out1 : Outport
  wires:
  Constant1/1 -> Switch/2
  Constant/1 -> Switch/1
  Switch/1 -> Out1/1
  In1/1 -> Switch/3

== system inp/INP/IMU/Subsystem2 ==
  In1 : Inport
  Constant : Constant  Value=KINP_MemOffsetAccX_raw16_ovrdval
  Constant1 : Constant  Value=KINP_MemOffsetAccX_raw16_ovrdflg
  Switch : Switch  Criteria=u2 ~= 0
  Out1 : Outport
  wires:
  Constant1/1 -> Switch/2
  Constant/1 -> Switch/1
  Switch/1 -> Out1/1
  In1/1 -> Switch/3

== system inp/INP/IMU/Subsystem3 ==
  In1 : Inport
  Constant : Constant  Value=KINP_MemOffsetGyroZ_raw16_ovrdval
  Constant1 : Constant  Value=KINP_MemOffsetGyroZ_raw16_ovrdflg
  Switch : Switch  Criteria=u2 ~= 0
  Out1 : Outport
  wires:
  Switch/1 -> Out1/1
  Constant/1 -> Switch/1
  Constant1/1 -> Switch/2
  In1/1 -> Switch/3

== system inp/INP/IMU/Subsystem4 ==
  In1 : Inport
  Constant : Constant  Value=KINP_MemOffsetAccZ_raw16_ovrdval
  Constant1 : Constant  Value=KINP_MemOffsetAccZ_raw16_ovrdflg
  Switch : Switch  Criteria=u2 ~= 0
  Out1 : Outport
  wires:
  Switch/1 -> Out1/1
  Constant/1 -> Switch/1
  Constant1/1 -> Switch/2
  In1/1 -> Switch/3

== system inp/INP/IMU/Subsystem5 ==
  In1 : Inport
  Constant : Constant  Value=KINP_MemOffsetAccY_raw16_ovrdval
  Constant1 : Constant  Value=KINP_MemOffsetAccY_raw16_ovrdflg
  Switch : Switch  Criteria=u2 ~= 0
  Out1 : Outport
  wires:
  Constant1/1 -> Switch/2
  Constant/1 -> Switch/1
  Switch/1 -> Out1/1
  In1/1 -> Switch/3

== system inp/INP/IMU/Subsystem6 ==
  In1 : Inport
  Constant : Constant  Value=KINP_SensingGyroY_raw16_ovrdval
  Constant1 : Constant  Value=KINP_SensingGyroY_raw16_ovrdflg
  Switch : Switch  Criteria=u2 ~= 0
  Out1 : Outport
  wires:
  Constant1/1 -> Switch/2
  Constant/1 -> Switch/1
  Switch/1 -> Out1/1
  In1/1 -> Switch/3

== system inp/INP/IMU/Subsystem7 ==
  In1 : Inport
  Constant : Constant  Value=KINP_SensingGyroX_raw16_ovrdval
  Constant1 : Constant  Value=KINP_SensingGyroX_raw16_ovrdflg
  Switch : Switch  Criteria=u2 ~= 0
  Out1 : Outport
  wires:
  Switch/1 -> Out1/1
  Constant/1 -> Switch/1
  Constant1/1 -> Switch/2
  In1/1 -> Switch/3

== system inp/INP/IMU/Subsystem8 ==
  In1 : Inport
  Constant : Constant  Value=KINP_SensingAccX_raw16_ovrdval
  Constant1 : Constant  Value=KINP_SensingAccX_raw16_ovrdflg
  Switch : Switch  Criteria=u2 ~= 0
  Out1 : Outport
  wires:
  Switch/1 -> Out1/1
  Constant/1 -> Switch/1
  Constant1/1 -> Switch/2
  In1/1 -> Switch/3

== system inp/INP/IMU/Subsystem9 ==
  In1 : Inport
  Constant : Constant  Value=KINP_SensingGyroZ_raw16_ovrdval
  Constant1 : Constant  Value=KINP_SensingGyroZ_raw16_ovrdflg
  Switch : Switch  Criteria=u2 ~= 0
  Out1 : Outport
  wires:
  Constant1/1 -> Switch/2
  Constant/1 -> Switch/1
  Switch/1 -> Out1/1
  In1/1 -> Switch/3
